simulink model "Simulink_TEP"  (R2024a)
settings: Solver=FixedStepAuto  StartTime=0.0  StopTime=5  FixedStep=1/3600  RelTol=1e-3
model workspace (MAT data in the model file):
  AD : Simulink.Parameter (value not decoded)
  AG : Simulink.Parameter (value not decoded)
  AH : Simulink.Parameter (value not decoded)
  AV : Simulink.Parameter (value not decoded)
  AVP : Simulink.Parameter (value not decoded)
  BCHL : Simulink.Parameter (value not decoded)
  BCHV : Simulink.Parameter (value not decoded)
  BD : Simulink.Parameter (value not decoded)
  BG : Simulink.Parameter (value not decoded)
  BH : Simulink.Parameter (value not decoded)
  BVP : Simulink.Parameter (value not decoded)
  CD : Simulink.Parameter (value not decoded)
  CG : Simulink.Parameter (value not decoded)
  CH : Simulink.Parameter (value not decoded)
  CVP : Simulink.Parameter (value not decoded)
  XMW : Simulink.Parameter (value not decoded)
symbols that are objects in the model workspace (value not decoded): AD, AG, AH, AV, AVP, BD, BG, BH, BVP, CD, CG, CH, CVP, XMW
undefined symbols (not defined in the file or in its folder): magnitude, SETPT, XMEAS, XMV
libraries: mylib x165, dspindex x17
(part 8 of 10)

== system Simulink_TEP/Random number generator/Disturbances I=10-12/TESUB7(11)/Subsystem ==
  In2 : Inport
  G : Inport  Port=2
  If Action Subsystem : Subsystem  TreatAsAtomicUnit=on
  If Action Subsystem1 : Subsystem  TreatAsAtomicUnit=on
  If5 : If  IfExpression=u1 == 0
  Merge : Merge
  G1 : Outport  VectorParamsAs1DForOutWhenUnconnected=off
  wires:
  In2/1 -> If Action Subsystem1/1(In1), If5/1
  If5/2 -> If Action Subsystem1/Action
  If Action Subsystem1/1(Out1) -> Merge/1
  If5/1 -> If Action Subsystem/Action
  If Action Subsystem/1(Out1) -> Merge/2
  G/1 -> If Action Subsystem/1(In1)
  Merge/1 -> G1/1

== system Simulink_TEP/Random number generator/Disturbances I=10-12/TESUB7(11)/TNEXT(11) ==
  Bus Selector : BusSelector  OutputSignals=TNEXT
  Clock3 : Clock
  If3 : If  NumInputs=3  IfExpression=u1 ~= 0 & u1 >= u2 & u3 < 0.1  ShowElse=off
  IF(11) : Outport  VectorParamsAs1DForOutWhenUnconnected=off
  wires:
  Bus Selector/1 -> If3/2  "<TNEXT>"
  Clock3/1 -> If3/1
  If3/1 -> IF(11)/1
  [DIST11] -> Bus Selector/1
  [SWLK_11] -> If3/3

== system Simulink_TEP/Random number generator/Disturbances I=10-12/TESUB7(12)/If Action Subsystem3 ==
  G : Inport
  Action Port : ActionPort  ActionPortLabel=if(u1 ~= 0 & u1 >= u2 & u3 < 0.1)
  Constant : Constant  Value=-1
  TESUB7 G-New : mylib/TESUB7 G-New  SystemSampleTime=-1  VariantActivationTime=update diagram  AllowFlexibleInterface=on  Latency=0  AutoFrameSizeCalculation=off
  TESUB7(12) : Outport  VectorParamsAs1DForOutWhenUnconnected=off
  G_NEW : Outport  Port=2  OutputWhenDisabled=reset  InitialOutput=[0]  VectorParamsAs1DForOutWhenUnconnected=off
  wires:
  Constant/1 -> TESUB7 G-New/1
  G/1 -> TESUB7 G-New/2
  TESUB7 G-New/2 -> G_NEW/1
  TESUB7 G-New/1 -> TESUB7(12)/1

== system Simulink_TEP/Random number generator/Disturbances I=10-12/TESUB7(12)/Subsystem ==
  In2 : Inport
  G : Inport  Port=2
  If Action Subsystem : Subsystem  TreatAsAtomicUnit=on
  If Action Subsystem1 : Subsystem  TreatAsAtomicUnit=on
  If5 : If  IfExpression=u1 == 0
  Merge : Merge
  G1 : Outport  VectorParamsAs1DForOutWhenUnconnected=off
  wires:
  In2/1 -> If Action Subsystem1/1(In1), If5/1
  If5/2 -> If Action Subsystem1/Action
  If Action Subsystem1/1(Out1) -> Merge/1
  If5/1 -> If Action Subsystem/Action
  If Action Subsystem/1(Out1) -> Merge/2
  G/1 -> If Action Subsystem/1(In1)
  Merge/1 -> G1/1

== system Simulink_TEP/Random number generator/Disturbances I=10-12/TESUB7(12)/TNEXT(12) ==
  Bus Selector : BusSelector  OutputSignals=TNEXT
  Clock3 : Clock
  If3 : If  NumInputs=3  IfExpression=u1 ~= 0 & u1 >= u2 & u3 < 0.1  ShowElse=off
  IF(12) : Outport  VectorParamsAs1DForOutWhenUnconnected=off
  wires:
  Bus Selector/1 -> If3/2  "<TNEXT>"
  Clock3/1 -> If3/1
  If3/1 -> IF(12)/1
  [DIST12] -> Bus Selector/1
  [SWLK_12] -> If3/3

== system Simulink_TEP/Random number generator/Process Measurements XMEAS(I) I=1-22/If Action Subsystem3/Subsystem ==
  G : Inport
  Bus Creator : BusCreator  Inputs=5
  Bus Creator1 : BusCreator  Inputs=5
  Bus Creator2 : BusCreator  Inputs=4
  Bus Creator3 : BusCreator  Inputs=5
  Bus Creator4 : BusCreator  Inputs=7
  Subsystem : Subsystem
  Subsystem1 : Subsystem
  Subsystem2 : Subsystem
  Subsystem3 : Subsystem
  XMNS : Outport  VectorParamsAs1DForOutWhenUnconnected=off
  G_NEW : Outport  Port=2  VectorParamsAs1DForOutWhenUnconnected=off
  wires:
  G/1 -> Subsystem/1(G)
  Subsystem/1(XMNS(1)) -> Bus Creator/1
  Subsystem/2(XMNS(2)) -> Bus Creator/2
  Subsystem/3(XMNS(3)) -> Bus Creator/3
  Subsystem/4(XMNS(4)) -> Bus Creator/4
  Subsystem/5(XMNS(5)) -> Bus Creator/5
  Subsystem/6(G_NEW) -> Subsystem1/1(G)
  Subsystem1/6(G_NEW) -> Subsystem2/1(G)
  Subsystem1/2(XMNS(7)) -> Bus Creator1/2
  Subsystem1/3(XMNS(8)) -> Bus Creator1/3
  Subsystem1/4(XMNS(9)) -> Bus Creator1/4
  Subsystem1/1(XMNS(6)) -> Bus Creator1/1
  Subsystem1/5(XMNS(10)) -> Bus Creator1/5
  Bus Creator1/1 -> Bus Creator2/2
  Bus Creator2/1 -> XMNS/1
  Bus Creator/1 -> Bus Creator2/1
  Subsystem2/1(XMNS(11)) -> Bus Creator3/1
  Bus Creator3/1 -> Bus Creator2/3
  Subsystem2/4(XMNS(14)) -> Bus Creator3/4
  Subsystem2/5(XMNS(15)) -> Bus Creator3/5
  Subsystem2/2(XMNS(12)) -> Bus Creator3/2
  Subsystem2/3(XMNS(13)) -> Bus Creator3/3
  Subsystem2/6(G_NEW) -> Subsystem3/1(G)
  Subsystem3/2(XMNS(17)) -> Bus Creator4/2
  Subsystem3/3(XMNS(18)) -> Bus Creator4/3
  Subsystem3/4(XMNS(19)) -> Bus Creator4/4
  Bus Creator4/1 -> Bus Creator2/4
  Subsystem3/5(XMNS(20)) -> Bus Creator4/5
  Subsystem3/8(G_NEW) -> G_NEW/1
  Subsystem3/1(XMNS(16)) -> Bus Creator4/1
  Subsystem3/6(XMNS(21)) -> Bus Creator4/6
  Subsystem3/7(XMNS(22)) -> Bus Creator4/7

== system Simulink_TEP/Random number generator/Process Measurements XMEAS(I) I=1-22/Subsystem/If Action Subsystem ==
  In1 : Inport
  Action Port : ActionPort  ActionPortLabel=if(u1 == 0)
  Out1 : Outport  VectorParamsAs1DForOutWhenUnconnected=off
  wires:
  In1/1 -> Out1/1

== system Simulink_TEP/Random number generator/Process Measurements XMEAS(I) I=1-22/Subsystem/If Action Subsystem1 ==
  In1 : Inport
  Action Port : ActionPort  ActionPortLabel=else
  Out1 : Outport  VectorParamsAs1DForOutWhenUnconnected=off
  wires:
  In1/1 -> Out1/1

== system Simulink_TEP/Random number generator/Process Measurements XMEAS(I) I=23-36/If Action Subsystem3/Subsystem ==
  G : Inport
  Bus Creator : BusCreator  Inputs=5
  Bus Creator1 : BusCreator  Inputs=5
  Bus Creator2 : BusCreator  Inputs=3
  Bus Creator3 : BusCreator  Inputs=4
  Subsystem : Subsystem
  Subsystem1 : Subsystem
  Subsystem2 : Subsystem
  XMNS : Outport  VectorParamsAs1DForOutWhenUnconnected=off
  G_NEW : Outport  Port=2  VectorParamsAs1DForOutWhenUnconnected=off
  wires:
  G/1 -> Subsystem/1(G)
  Subsystem/1(XMNS(23)) -> Bus Creator/1
  Subsystem/2(XMNS(24)) -> Bus Creator/2
  Subsystem/3(XMNS(25)) -> Bus Creator/3
  Subsystem/4(XMNS(26)) -> Bus Creator/4
  Subsystem/5(XMNS(27)) -> Bus Creator/5
  Subsystem/6(G_NEW) -> Subsystem1/1(G)
  Subsystem1/6(G_NEW) -> Subsystem2/1(G)
  Subsystem1/2(XMNS(29)) -> Bus Creator1/2
  Subsystem1/3(XMNS(30)) -> Bus Creator1/3
  Subsystem1/4(XMNS(31)) -> Bus Creator1/4
  Subsystem1/1(XMNS(28)) -> Bus Creator1/1
  Subsystem1/5(XMNS(32)) -> Bus Creator1/5
  Bus Creator1/1 -> Bus Creator2/2
  Bus Creator2/1 -> XMNS/1
  Bus Creator/1 -> Bus Creator2/1
  Subsystem2/1(XMNS(33)) -> Bus Creator3/1
  Bus Creator3/1 -> Bus Creator2/3
  Subsystem2/4(XMNS(36)) -> Bus Creator3/4
  Subsystem2/2(XMNS(34)) -> Bus Creator3/2
  Subsystem2/3(XMNS(35)) -> Bus Creator3/3
  Subsystem2/5(G_NEW) -> G_NEW/1

== system Simulink_TEP/Random number generator/Process Measurements XMEAS(I) I=23-36/Subsystem/If Action Subsystem ==
  In1 : Inport
  Action Port : ActionPort  ActionPortLabel=if(u1 == 0)
  Out1 : Outport  VectorParamsAs1DForOutWhenUnconnected=off
  wires:
  In1/1 -> Out1/1

== system Simulink_TEP/Random number generator/Process Measurements XMEAS(I) I=23-36/Subsystem/If Action Subsystem1 ==
  In1 : Inport
  Action Port : ActionPort  ActionPortLabel=else
  Out1 : Outport  VectorParamsAs1DForOutWhenUnconnected=off
  wires:
  In1/1 -> Out1/1

== system Simulink_TEP/Random number generator/Process Measurements XMEAS(I) I=37-41/If Action Subsystem3/Subsystem ==
  G : Inport
  Bus Creator : BusCreator  Inputs=5
  Subsystem : Subsystem
  XMNS : Outport  VectorParamsAs1DForOutWhenUnconnected=off
  G_NEW : Outport  Port=2  VectorParamsAs1DForOutWhenUnconnected=off
  wires:
  G/1 -> Subsystem/1(G)
  Subsystem/1(XMNS(37)) -> Bus Creator/1
  Subsystem/2(XMNS(38)) -> Bus Creator/2
  Subsystem/3(XMNS(39)) -> Bus Creator/3
  Subsystem/4(XMNS(40)) -> Bus Creator/4
  Subsystem/5(XMNS(41)) -> Bus Creator/5
  Bus Creator/1 -> XMNS/1
  Subsystem/6(G_NEW) -> G_NEW/1

== system Simulink_TEP/Random number generator/Process Measurements XMEAS(I) I=37-41/Subsystem/If Action Subsystem ==
  In1 : Inport
  Action Port : ActionPort  ActionPortLabel=if(u1 == 0)
  Out1 : Outport  VectorParamsAs1DForOutWhenUnconnected=off
  wires:
  In1/1 -> Out1/1

== system Simulink_TEP/Random number generator/Process Measurements XMEAS(I) I=37-41/Subsystem/If Action Subsystem1 ==
  In1 : Inport
  Action Port : ActionPort  ActionPortLabel=else
  Out1 : Outport  VectorParamsAs1DForOutWhenUnconnected=off
  wires:
  In1/1 -> Out1/1

== system Simulink_TEP/Reactor/Reaction Rates/Component reaction rate lb-mol//h/Subsystem ==
  RR : Inport
  " " : Sum  Inputs=---
  Bus Selector : BusSelector  OutputSignals=RR(1),RR(2),RR(3)
  CRXR(1) : Outport  VectorParamsAs1DForOutWhenUnconnected=off
  wires:
  " "/1 -> CRXR(1)/1  "CRXR(1)"
  Bus Selector/2 -> " "/2  "<RR(2)>"
  Bus Selector/3 -> " "/3  "<RR(3)>"
  RR/1 -> Bus Selector/1
  Bus Selector/1 -> " "/1  "<RR(1)>"

== system Simulink_TEP/Reactor/Reaction Rates/Component reaction rate lb-mol//h/Subsystem1 ==
  RR : Inport
  " " : Sum  Inputs=--
  Bus Selector : BusSelector  OutputSignals=RR(1),RR(2)
  CRXR(3) : Outport  VectorParamsAs1DForOutWhenUnconnected=off
  wires:
  " "/1 -> CRXR(3)/1  "CRXR(3)"
  RR/1 -> Bus Selector/1
  Bus Selector/1 -> " "/1  "<RR(1)>"
  Bus Selector/2 -> " "/2  "<RR(2)>"

== system Simulink_TEP/Reactor/Reaction Rates/Component reaction rate lb-mol//h/Subsystem2 ==
  RR : Inport
  " " : Sum  Inputs=--
  Bus Selector : BusSelector  OutputSignals=RR(1),RR(4)
  Gain : Gain  Gain=1.5
  CRXR(4) : Outport  VectorParamsAs1DForOutWhenUnconnected=off
  wires:
  Gain/1 -> " "/2
  Bus Selector/1 -> " "/1  "<RR(1)>"
  " "/1 -> CRXR(4)/1  "CRXR(4)"
  RR/1 -> Bus Selector/1
  Bus Selector/2 -> Gain/1  "<RR(4)>"

== system Simulink_TEP/Reactor/Reaction Rates/Component reaction rate lb-mol//h/Subsystem3 ==
  RR : Inport
  " " : Sum  Inputs=--
  Bus Selector : BusSelector  OutputSignals=RR(2),RR(3)
  CRXR(5) : Outport  VectorParamsAs1DForOutWhenUnconnected=off
  wires:
  " "/1 -> CRXR(5)/1  "CRXR(5)"
  RR/1 -> Bus Selector/1
  Bus Selector/1 -> " "/1  "<RR(2)>"
  Bus Selector/2 -> " "/2  "<RR(3)>"

== system Simulink_TEP/Reactor/Reaction Rates/Component reaction rate lb-mol//h/Subsystem4 ==
  RR : Inport
  " " : Sum
  Bus Selector : BusSelector  OutputSignals=RR(3),RR(4)
  CRXR(6) : Outport  VectorParamsAs1DForOutWhenUnconnected=off
  wires:
  " "/1 -> CRXR(6)/1  "CRXR(6)"
  RR/1 -> Bus Selector/1
  Bus Selector/2 -> " "/2  "<RR(4)>"
  Bus Selector/1 -> " "/1  "<RR(3)>"

== system Simulink_TEP/Reactor/Reaction Rates/Component reaction rate lb-mol//h/Subsystem5 ==
  RR : Inport
  Bus Selector : BusSelector  OutputSignals=RR(1)
  Gain : Gain
  CRXR(7) : Outport  VectorParamsAs1DForOutWhenUnconnected=off
  wires:
  Bus Selector/1 -> Gain/1  "<RR(1)>"
  RR/1 -> Bus Selector/1
  Gain/1 -> CRXR(7)/1  "CRXR(7)"

== system Simulink_TEP/Reactor/Reaction Rates/Component reaction rate lb-mol//h/Subsystem6 ==
  RR : Inport
  " " : Gain
  Bus Selector : BusSelector  OutputSignals=RR(2)
  CRXR(8) : Outport  VectorParamsAs1DForOutWhenUnconnected=off
  wires:
  " "/1 -> CRXR(8)/1  "CRXR(8)"
  RR/1 -> Bus Selector/1
  Bus Selector/1 -> " "/1  "<RR(2)>"

== system Simulink_TEP/Reactor/Reaction Rates/Reaction rates lb-mol//h/ Reaction rate of reaction 4 lb-mol//ft3·h     ==
  PPR : Inport
  TKR : Inport  Port=2
  Activation energy cal/mol : Constant  Value=60000
  Bus Selector : BusSelector  OutputSignals=PPR(1),PPR(4)
  Divide : Product  Inputs=*//
  Divide1 : Product  Inputs=3
  Gain : Gain  Gain=0.767488334
  Math Function2 : Math  SignedPower=on
  Preexponential factor lb-mol/ft3·h·mmHg : Constant  Value=53.4060443
  Subtract : Sum  Inputs=+-
  Universal gas constant cal/mol·K : Constant  Value=1.987
  RR(4) : Outport  VectorParamsAs1DForOutWhenUnconnected=off
  wires:
  Divide/1 -> Subtract/2
  Universal gas constant cal/mol·K/1 -> Divide/2
  Preexponential factor lb-mol/ft3·h·mmHg/1 -> Subtract/1
  Activation energy cal/mol/1 -> Divide/1
  TKR/1 -> Divide/3
  Subtract/1 -> Math Function2/1
  Divide1/1 -> RR(4)/1
  Bus Selector/2 -> Divide1/3  "<PPR(4)>"
  Gain/1 -> Divide1/1
  Math Function2/1 -> Gain/1
  PPR/1 -> Bus Selector/1
  Bus Selector/1 -> Divide1/2  "<PPR(1)>"

== system Simulink_TEP/Reactor/Reaction Rates/Reaction rates lb-mol//h/Reaction rate of reaction 1 lb-mol//ft3·h ==
  PPR : Inport
  TKR : Inport  Port=2
  " " : Constant  Value=0
  Abs : Abs  SaturateOnIntegerOverflow=off
  Bus Selector : BusSelector  OutputSignals=PPR(1),PPR(3)
  If : If  NumInputs=2  IfExpression=u1>0 & u2>0
  If Action Subsystem : Subsystem  TreatAsAtomicUnit=on
  If Action Subsystem2 : Subsystem  TreatAsAtomicUnit=on
  Merge1 : Merge
  "RR(1) Reaction rate of 1st reaction lb-mol/ft3·h " : Subsystem
  RR(1) : Outport  VectorParamsAs1DForOutWhenUnconnected=off
  wires:
  "RR(1) Reaction rate of 1st reaction lb-mol/ft3·h "/1(RR(1)) -> If Action Subsystem/1(In1)
  If/1 -> If Action Subsystem/Action
  " "/1 -> If Action Subsystem2/1(In1)
  If/2 -> If Action Subsystem2/Action
  Merge1/1 -> Abs/1
  If Action Subsystem/1(Out1) -> Merge1/1
  If Action Subsystem2/1(Out1) -> Merge1/2
  TKR/1 -> "RR(1) Reaction rate of 1st reaction lb-mol/ft3·h "/2(TKR)
  Abs/1 -> RR(1)/1
  PPR/1 -> "RR(1) Reaction rate of 1st reaction lb-mol/ft3·h "/1(PPR), Bus Selector/1
  Bus Selector/1 -> If/1  "<PPR(1)>"
  Bus Selector/2 -> If/2  "<PPR(3)>"

== system Simulink_TEP/Reactor/Reaction Rates/Reaction rates lb-mol//h/Reaction rate of reaction 2 lb-mol//ft3·h ==
  PPR : Inport
  TKR : Inport  Port=2
  " " : Constant  Value=0
  Abs : Abs  SaturateOnIntegerOverflow=off
  Bus Selector : BusSelector  OutputSignals=PPR(1),PPR(3)
  If : If  NumInputs=2  IfExpression=u1>0 & u2>0
  If Action Subsystem : Subsystem  TreatAsAtomicUnit=on
  If Action Subsystem2 : Subsystem  TreatAsAtomicUnit=on
  Merge1 : Merge
  "RR(2) Reaction rate of 2nd reaction lb-mol/ft3·h " : Subsystem
  RR(2) : Outport  VectorParamsAs1DForOutWhenUnconnected=off
  wires:
  If/1 -> If Action Subsystem/Action
  If/2 -> If Action Subsystem2/Action
  "RR(2) Reaction rate of 2nd reaction lb-mol/ft3·h "/1(RR(2)) -> If Action Subsystem/1(In1)
  " "/1 -> If Action Subsystem2/1(In1)
  If Action Subsystem2/1(Out1) -> Merge1/2
  TKR/1 -> "RR(2) Reaction rate of 2nd reaction lb-mol/ft3·h "/2(TKR)
  If Action Subsystem/1(Out1) -> Merge1/1
  Merge1/1 -> Abs/1
  Abs/1 -> RR(2)/1
  PPR/1 -> "RR(2) Reaction rate of 2nd reaction lb-mol/ft3·h "/1(PPR), Bus Selector/1
  Bus Selector/1 -> If/1  "<PPR(1)>"
  Bus Selector/2 -> If/2  "<PPR(3)>"

== system Simulink_TEP/Reactor/Reaction Rates/Reaction rates lb-mol//h/Reaction rate of reaction 3 lb-mol//ft3·h   ==
  PPR : Inport
  TKR : Inport  Port=2
  Activation energy cal/mol : Constant  Value=60000
  Bus Selector : BusSelector  OutputSignals=PPR(1),PPR(5)
  Divide : Product  Inputs=*//
  Divide1 : Product  Inputs=3
  Math Function2 : Math  SignedPower=on
  Preexponential factor lb-mol/ft3·h·mmHg : Constant  Value=53.4060443
  Subtract : Sum  Inputs=+-
  Universal gas constant cal/mol·K : Constant  Value=1.987
  RR(3) : Outport  VectorParamsAs1DForOutWhenUnconnected=off
  wires:
  Divide/1 -> Subtract/2
  Universal gas constant cal/mol·K/1 -> Divide/2
  Preexponential factor lb-mol/ft3·h·mmHg/1 -> Subtract/1
  Activation energy cal/mol/1 -> Divide/1
  TKR/1 -> Divide/3
  Subtract/1 -> Math Function2/1
  Bus Selector/2 -> Divide1/3  "<PPR(5)>"
  Divide1/1 -> RR(3)/1
  Math Function2/1 -> Divide1/1
  PPR/1 -> Bus Selector/1
  Bus Selector/1 -> Divide1/2  "<PPR(1)>"

== system Simulink_TEP/Reactor/Reactor Heat exchanger/Position of Valve 12 %/Control valve ==
  XMV(12) : Inport
  Valve opening limits : mylib/Valve opening limits  SystemSampleTime=-1  VariantActivationTime=update diagram  AllowFlexibleInterface=on  Latency=0  AutoFrameSizeCalculation=off
  VCV(12) : Outport  PortDimensions=1  VectorParamsAs1DForOutWhenUnconnected=off
  wires:
  Valve opening limits/1 -> VCV(12)/1
  XMV(12)/1 -> Valve opening limits/1

== system Simulink_TEP/Reactor/Reactor Heat exchanger/Reactor Heat exchanger/AGSP Agitation speed ==
  VPOS(12) : Inport
  " " : Product  Inputs=*/
  Add : Sum
  Constant1 : Constant  Value=150
  Constant2 : Constant  Value=100
  AGSP : Outport  VectorParamsAs1DForOutWhenUnconnected=off
  wires:
  Constant2/1 -> " "/2
  " "/1 -> AGSP/1
  VPOS(12)/1 -> Add/1
  Constant1/1 -> Add/2
  Add/1 -> " "/1

== system Simulink_TEP/Reactor/Reactor Heat exchanger/Reactor Heat exchanger/FWR Flow of cooling water to reactor lb-mol//h ==
  VPOS(10) : Inport
  VRNG(10) : Inport  Port=2
  " " : Product  Inputs=**/
  Constant2 : Constant  Value=100
  FWR : Outport  VectorParamsAs1DForOutWhenUnconnected=off
  wires:
  Constant2/1 -> " "/3
  " "/1 -> FWR/1
  VPOS(10)/1 -> " "/1
  VRNG(10)/1 -> " "/2

== system Simulink_TEP/Reactor/Reactor Heat exchanger/Reactor Heat exchanger/Subsystem ==
  VLR : Inport
  Constant : Constant  Value=7.8
  Constant1 : Constant
  Constant2 : Constant  Value=0
  Constant3 : Constant  Value=0.025
  Constant4 : Constant  Value=0.25
  Divide : Product  Inputs=*/
  Divide1 : Product  Inputs=**
  If : If  IfExpression=u1 > 50  ElseIfExpressions=u1 < 10
  If Action Subsystem : Subsystem  TreatAsAtomicUnit=on
  If Action Subsystem1 : Subsystem  TreatAsAtomicUnit=on
  If Action Subsystem2 : Subsystem  TreatAsAtomicUnit=on
  Subtract : Sum  Inputs=+-
  UARLEV : Merge  Inputs=3
  "UARLEV " : Outport  VectorParamsAs1DForOutWhenUnconnected=off
  wires:
  If/2 -> If Action Subsystem1/Action
  If/1 -> If Action Subsystem/Action
  UARLEV/1 -> "UARLEV "/1
  If Action Subsystem1/1(Out1) -> UARLEV/2
  If Action Subsystem/1(Out1) -> UARLEV/1
  If/3 -> If Action Subsystem2/Action
  If Action Subsystem2/1(Out1) -> UARLEV/3
  VLR/1 -> Divide/1
  Constant/1 -> Divide/2
  Divide/1 -> Divide1/2, If/1
  Constant1/1 -> If Action Subsystem/1(In1)
  Constant2/1 -> If Action Subsystem1/1(In1)
  Constant3/1 -> Divide1/1
  Divide1/1 -> Subtract/1
  Constant4/1 -> Subtract/2
  Subtract/1 -> If Action Subsystem2/1(In1)

== system Simulink_TEP/Reactor/Reactor Heat exchanger/Reactor Heat exchanger/Subsystem1 ==
  FWR : Inport
  QUR : Inport  Port=2  PortDimensions=1
  Constant1 : Constant  Value=1e6
  Constant2 : Constant  Value=1.8
  Constant6 : Constant  Value=500.53
  Divide : Product  Inputs=*/
  Divide1 : Product
  Divide2 : Product  Inputs=*/
  HWR : Constant  Value=7060
  Product : Product  Inputs=3
  Subtract : Sum  Inputs=+-
  TCWR : Subsystem
  TCWR-TWR : Sum  Inputs=+-
  YP(37) : Integrator  InitialConditionSource=external
  YY(37) : Constant  Value=94.59927549
  "YY(37) " : Outport  VectorParamsAs1DForOutWhenUnconnected=off
  tag scope: TWR=global
  wires:
  Divide2/1 -> YP(37)/1
  YY(37)/1 -> YP(37)/2
  TCWR/1(TCWR) -> TCWR-TWR/1
  YP(37)/1 -> [TWR], "YY(37) "/1, TCWR-TWR/2
  FWR/1 -> Product/1
  Constant6/1 -> Product/2
  TCWR-TWR/1 -> Product/3
  QUR/1 -> Divide1/1
  Constant1/1 -> Divide1/2
  Divide1/1 -> Divide/1
  Constant2/1 -> Divide/2
  Product/1 -> Subtract/1
  Divide/1 -> Subtract/2
  Subtract/1 -> Divide2/1
  HWR/1 -> Divide2/2

== system Simulink_TEP/Reactor/Stream 8/Subsystem/If Action Subsystem ==
  In1 : Inport
  Action Port : ActionPort  ActionPortLabel=if(u1 < 0)
  Out1 : Outport  VectorParamsAs1DForOutWhenUnconnected=off
  wires:
  In1/1 -> Out1/1

== system Simulink_TEP/Reactor/Stream 8/Subsystem/If Action Subsystem1 ==
  In1 : Inport
  Action Port : ActionPort  ActionPortLabel=else
  Out1 : Outport  VectorParamsAs1DForOutWhenUnconnected=off
  wires:
  In1/1 -> Out1/1

== system Simulink_TEP/Reactor/Volume of Reactor/DLR Molar Density of Liquids in Reactor lb-mol//ft³    /DLR Molar Density of Liquids in Reactor lb-mol//ft³  ==
  X : Inport
  T : Inport  Port=2
  "  " : Constant
  "    " : Product  Inputs=*/
  AD(I) : Constant  Value=AD
  Add2 : Sum
  BD(I) : Constant  Value=BD
  CD(I) : Constant  Value=CD
  Liquid Density of Components lb/ft³ : Sum
  Molecular weight of components lb/lb-mol : Constant  Value=XMW
  Product : Product
  Product1 : Product
  Product2 : Product
  Sum of Elements : Sum  Inputs=+
  V Molar Volume of Components ft³/lb-mol : Product  Inputs=*/
  "R " : Outport  VectorParamsAs1DForOutWhenUnconnected=off
  wires:
  Liquid Density of Components lb/ft³/1 -> V Molar Volume of Components ft³/lb-mol/2
  Product1/1 -> Liquid Density of Components lb/ft³/2
  T/1 -> Product1/2, Product/2
  "  "/1 -> "    "/1
  AD(I)/1 -> Liquid Density of Components lb/ft³/1
  Add2/1 -> Product1/1
  V Molar Volume of Components ft³/lb-mol/1 -> Sum of Elements/1
  CD(I)/1 -> Product/1
  Product2/1 -> V Molar Volume of Components ft³/lb-mol/1
  BD(I)/1 -> Add2/1
  Product/1 -> Add2/2
  "    "/1 -> "R "/1
  X/1 -> Product2/1
  Sum of Elements/1 -> "    "/2
  Molecular weight of components lb/lb-mol/1 -> Product2/2

== system Simulink_TEP/Separator/Stream 10/Subsystem/If Action Subsystem ==
  In1 : Inport
  Action Port : ActionPort  ActionPortLabel=if(u1 < 0)
  Out1 : Outport  VectorParamsAs1DForOutWhenUnconnected=off
  wires:
  In1/1 -> Out1/1

== system Simulink_TEP/Separator/Stream 10/Subsystem/If Action Subsystem1 ==
  In1 : Inport
  Action Port : ActionPort  ActionPortLabel=else
  Out1 : Outport  VectorParamsAs1DForOutWhenUnconnected=off
  wires:
  In1/1 -> Out1/1

== system Simulink_TEP/Separator/Stream 9/Subsystem/If Action Subsystem2 ==
  In1 : Inport
  Action Port : ActionPort  ActionPortLabel=if(u1 < 1E-3)
  Out1 : Outport  VectorParamsAs1DForOutWhenUnconnected=off
  wires:
  In1/1 -> Out1/1

== system Simulink_TEP/Separator/Stream 9/Subsystem/If Action Subsystem3 ==
  In1 : Inport
  Action Port : ActionPort  ActionPortLabel=else
  Out1 : Outport  PortDimensions=1  VectorParamsAs1DForOutWhenUnconnected=off
  wires:
  In1/1 -> Out1/1

== system Simulink_TEP/Separator/Stream 9/Subsystem/Pressure drop ==
  Constant : Constant  Value=0.0
  DLP : Sum  Inputs=+-
  DLP Pressure drop between separator and reactor : Merge
  If : If  IfExpression=u1 < 0
  If Action Subsystem : Subsystem  TreatAsAtomicUnit=on
  If Action Subsystem1 : Subsystem  TreatAsAtomicUnit=on
  Out1 : Outport  VectorParamsAs1DForOutWhenUnconnected=off
  wires:
  DLP Pressure drop between separator and reactor/1 -> Out1/1
  [PTV] -> DLP/1
  Constant/1 -> If Action Subsystem/1(In1)
  DLP/1 -> If Action Subsystem1/1(In1), If/1
  If/2 -> If Action Subsystem1/Action
  If/1 -> If Action Subsystem/Action
  [PTS] -> DLP/2
  If Action Subsystem1/1(Out1) -> DLP Pressure drop between separator and reactor/2
  If Action Subsystem/1(Out1) -> DLP Pressure drop between separator and reactor/1

== system Simulink_TEP/Separator/Volume of Separator/DLS Molar Density of Liquids in Reactor lb-mol//ft³    /DLS Molar Density of Liquids in Separator lb-mol//ft³  ==
  X : Inport
  T : Inport  Port=2
  "  " : Constant
  "    " : Product  Inputs=*/
  AD(I) : Constant  Value=AD
  Add2 : Sum
  BD(I) : Constant  Value=BD
  CD(I) : Constant  Value=CD
  Display : Display
  Display1 : Display
  Display2 : Display
  Liquid Density of Components lb/ft³ : Sum
  Product : Product
  Product1 : Product
  Product2 : Product
  Sum of Elements : Sum  Inputs=+
  V Molar Volume of Components ft³/lb-mol : Product  Inputs=*/
  XMW : Constant  Value=XMW
  "R " : Outport  VectorParamsAs1DForOutWhenUnconnected=off
  wires:
  Liquid Density of Components lb/ft³/1 -> V Molar Volume of Components ft³/lb-mol/2
  Product1/1 -> Liquid Density of Components lb/ft³/2
  T/1 -> Display/1, Product1/2, Product/2
  "  "/1 -> "    "/1
  AD(I)/1 -> Liquid Density of Components lb/ft³/1
  Add2/1 -> Product1/1
  V Molar Volume of Components ft³/lb-mol/1 -> Sum of Elements/1
  CD(I)/1 -> Product/1
  Product2/1 -> V Molar Volume of Components ft³/lb-mol/1
  BD(I)/1 -> Add2/1
  Product/1 -> Add2/2
  "    "/1 -> Display1/1, "R "/1
  X/1 -> Display2/1, Product2/1
  Sum of Elements/1 -> "    "/2
  XMW/1 -> Product2/2

== system Simulink_TEP/Stripper/Split Fractions/Split fraction/If Action Subsystem ==
  In1 : Inport
  Action Port : ActionPort  ActionPortLabel=if(u1 >0.1)
  Out1 : Outport  VectorParamsAs1DForOutWhenUnconnected=off
  wires:
  In1/1 -> Out1/1

== system Simulink_TEP/Stripper/Split Fractions/Split fraction/If Action Subsystem1 ==
  In1 : Inport
  Action Port : ActionPort  ActionPortLabel=if(u1 >170)
  Out1 : Outport  VectorParamsAs1DForOutWhenUnconnected=off
  wires:
  In1/1 -> Out1/1

== system Simulink_TEP/Stripper/Split Fractions/Split fraction/If Action Subsystem2 ==
  In1 : Inport
  Action Port : ActionPort  ActionPortLabel=elseif(u1<5.292)
  Out1 : Outport  VectorParamsAs1DForOutWhenUnconnected=off
  wires:
  In1/1 -> Out1/1

== system Simulink_TEP/Stripper/Split Fractions/Split fraction/If Action Subsystem3 ==
  In1 : Inport
  Action Port : ActionPort  ActionPortLabel=else
  Out1 : Outport  VectorParamsAs1DForOutWhenUnconnected=off
  wires:
  In1/1 -> Out1/1

== system Simulink_TEP/Stripper/Split Fractions/Split fraction/If Action Subsystem4 ==
  In1 : Inport
  Action Port : ActionPort  ActionPortLabel=else
  Out1 : Outport  VectorParamsAs1DForOutWhenUnconnected=off
  wires:
  In1/1 -> Out1/1

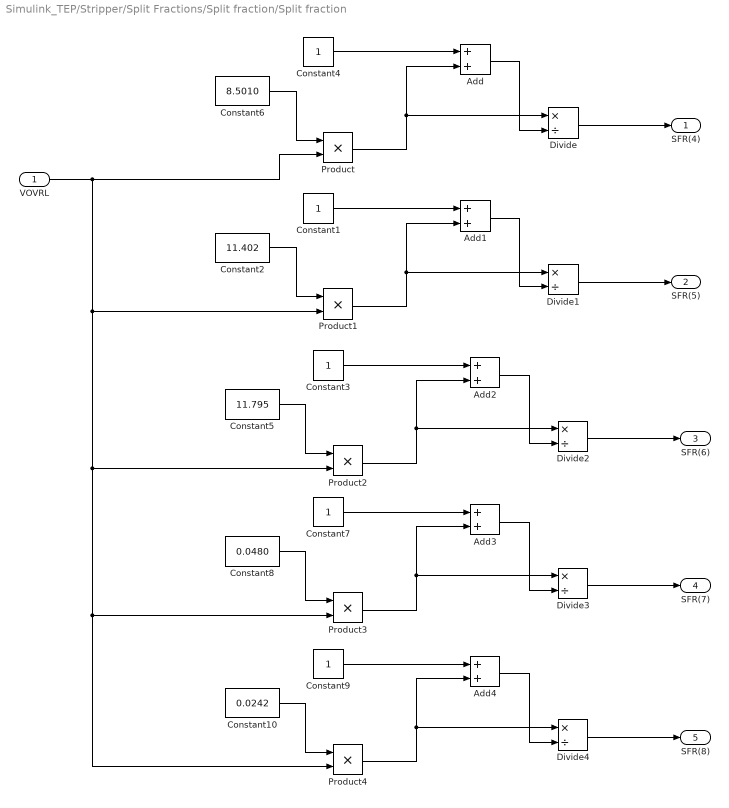
== system Simulink_TEP/Stripper/Split Fractions/Split fraction/Split fraction ==
  VOVRL : Inport
  Add{,1..4} (5 alike) : Sum
  Constant{1,3..4,7,9} (5 alike) : Constant
  Constant10 : Constant  Value=0.0242
  Constant2 : Constant  Value=11.402
  Constant5 : Constant  Value=11.795
  Constant6 : Constant  Value=8.5010
  Constant8 : Constant  Value=0.0480
  Divide{,1..4} (5 alike) : Product  Inputs=*/
  Product{,1..4} (5 alike) : Product
  SFR(4) : Outport  PortDimensions=1  VectorParamsAs1DForOutWhenUnconnected=off
  SFR(5) : Outport  Port=2  PortDimensions=1  VectorParamsAs1DForOutWhenUnconnected=off
  SFR(6) : Outport  Port=3  PortDimensions=1  VectorParamsAs1DForOutWhenUnconnected=off
  SFR(7) : Outport  Port=4  PortDimensions=1  VectorParamsAs1DForOutWhenUnconnected=off
  SFR(8) : Outport  Port=5  PortDimensions=1  VectorParamsAs1DForOutWhenUnconnected=off
  wires:
  Add/1 -> Divide/2
  Product/1 -> Divide/1, Add/2
  Constant4/1 -> Add/1
  Constant6/1 -> Product/1
  Divide/1 -> SFR(4)/1
  Product1/1 -> Divide1/1, Add1/2
  Add1/1 -> Divide1/2
  Constant1/1 -> Add1/1
  Constant2/1 -> Product1/1
  Divide1/1 -> SFR(5)/1
  Divide2/1 -> SFR(6)/1
  Product2/1 -> Divide2/1, Add2/2
  Add2/1 -> Divide2/2
  Constant3/1 -> Add2/1
  Constant5/1 -> Product2/1
  Divide3/1 -> SFR(7)/1
  Product3/1 -> Divide3/1, Add3/2
  Add3/1 -> Divide3/2
  Constant7/1 -> Add3/1
  Constant8/1 -> Product3/1
  Divide4/1 -> SFR(8)/1
  Product4/1 -> Divide4/1, Add4/2
  VOVRL/1 -> Product4/2, Product3/2, Product2/2, Product1/2, Product/2
  Add4/1 -> Divide4/2
  Constant9/1 -> Add4/1
  Constant10/1 -> Product4/1

== system Simulink_TEP/Stripper/Volume of Stripper/DLC Molar Density of Liquids in Stripper lb-mol//ft³    /DLC Molar Density of Liquids in Stripper lb-mol//ft³  ==
  X : Inport
  T : Inport  Port=2
  "  " : Constant
  "    " : Product  Inputs=*/
  AD(I) : Constant  Value=AD
  Add2 : Sum
  BD(I) : Constant  Value=BD
  CD(I) : Constant  Value=CD
  Constant : Constant  Value=XMW
  Liquid Density of Components lb/ft³ : Sum
  Product : Product
  Product1 : Product
  Product2 : Product
  Sum of Elements : Sum  Inputs=+
  V Molar Volume of Components ft³/lb-mol : Product  Inputs=*/
  "R " : Outport  VectorParamsAs1DForOutWhenUnconnected=off
  wires:
  Liquid Density of Components lb/ft³/1 -> V Molar Volume of Components ft³/lb-mol/2
  Product1/1 -> Liquid Density of Components lb/ft³/2
  T/1 -> Product1/2, Product/2
  "  "/1 -> "    "/1
  AD(I)/1 -> Liquid Density of Components lb/ft³/1
  Add2/1 -> Product1/1
  V Molar Volume of Components ft³/lb-mol/1 -> Sum of Elements/1
  CD(I)/1 -> Product/1
  Product2/1 -> V Molar Volume of Components ft³/lb-mol/1
  BD(I)/1 -> Add2/1
  Product/1 -> Add2/2
  "    "/1 -> "R "/1
  X/1 -> Product2/1
  Sum of Elements/1 -> "    "/2
  Constant/1 -> Product2/2

== system Simulink_TEP/Subsystem/Braatz/ /CONTROL 1 ==
  XMEAS(2) : Inport
  SETPT(1) : Inport  Port=2
  Constant1 : Constant  Value=GAIN1
  Constant2 : Constant  Value=HIGH1
  Constant3 : Constant  Value=SI1
  P Control : mylib/Braatz Control/P Control  SystemSampleTime=-1  VariantActivationTime=update diagram  AllowFlexibleInterface=on  Latency=0  AutoFrameSizeCalculation=off
  Sampling interval : mylib/Braatz Control/Sampling interval  SystemSampleTime=-1  VariantActivationTime=update diagram  AllowFlexibleInterface=on  Latency=0  AutoFrameSizeCalculation=off
  Unit Delay : UnitDelay  InitialCondition=XMV1_0  SampleTime=-1  HasFrameUpgradeWarning=on
  Unit Delay1 : UnitDelay  SampleTime=-1  HasFrameUpgradeWarning=on
  XMV(1) : Outport  VectorParamsAs1DForOutWhenUnconnected=off
  wires:
  Constant2/1 -> P Control/5
  Constant1/1 -> P Control/3
  SETPT(1)/1 -> P Control/1
  Unit Delay/1 -> P Control/2
  XMEAS(2)/1 -> P Control/4
  P Control/1 -> XMV(1)/1, Unit Delay/1
  Sampling interval/1 -> P Control/Action
  Constant3/1 -> Sampling interval/1
  Unit Delay1/1 -> P Control/6
  P Control/2 -> Unit Delay1/1

== system Simulink_TEP/Subsystem/Braatz/ /CONTROL 14 ==
  XMEAS(26) : Inport
  Constant : Constant  Value=SETPT14
  Constant1 : Constant  Value=GAIN14
  Constant2 : Constant  Value=TAUI14
  Constant3 : Constant  Value=HIGH14
  Constant5 : Constant  Value=SI14
  Constant6 : Constant  Value=HIGH1
  PI Control Setpoint : mylib/Braatz Control/PI Control Setpoint  SystemSampleTime=-1  VariantActivationTime=update diagram  AllowFlexibleInterface=on  Latency=0  AutoFrameSizeCalculation=off
  Sampling interval : mylib/Braatz Control/Sampling interval  SystemSampleTime=-1  VariantActivationTime=update diagram  AllowFlexibleInterface=on  Latency=0  AutoFrameSizeCalculation=off
  Unit Delay : UnitDelay  InitialCondition=SETPT1  SampleTime=-1  HasFrameUpgradeWarning=on
  Unit Delay1 : UnitDelay  SampleTime=-1  HasFrameUpgradeWarning=on
  SETPT(1) : Outport  VectorParamsAs1DForOutWhenUnconnected=off
  wires:
  Sampling interval/1 -> PI Control Setpoint/Action
  Constant/1 -> PI Control Setpoint/1
  XMEAS(26)/1 -> PI Control Setpoint/2
  PI Control Setpoint/1 -> SETPT(1)/1, Unit Delay/1
  Constant2/1 -> PI Control Setpoint/8
  Constant5/1 -> PI Control Setpoint/7, Sampling interval/1
  Constant1/1 -> PI Control Setpoint/6
  Constant3/1 -> PI Control Setpoint/3
  Unit Delay/1 -> PI Control Setpoint/4
  Constant6/1 -> PI Control Setpoint/5
  PI Control Setpoint/2 -> Unit Delay1/1
  Unit Delay1/1 -> PI Control Setpoint/9

== system Simulink_TEP/Subsystem/Braatz/ 1/CONTROL 15 ==
  XMEAS(27) : Inport
  Constant : Constant  Value=SETPT15
  Constant1 : Constant  Value=GAIN15
  Constant2 : Constant  Value=TAUI15
  Constant3 : Constant  Value=HIGH15
  Constant5 : Constant  Value=SI15
  Constant6 : Constant  Value=HIGH2
  PI Control Setpoint : mylib/Braatz Control/PI Control Setpoint  SystemSampleTime=-1  VariantActivationTime=update diagram  AllowFlexibleInterface=on  Latency=0  AutoFrameSizeCalculation=off
  Sampling interval : mylib/Braatz Control/Sampling interval  SystemSampleTime=-1  VariantActivationTime=update diagram  AllowFlexibleInterface=on  Latency=0  AutoFrameSizeCalculation=off
  Unit Delay : UnitDelay  InitialCondition=SETPT2  SampleTime=-1  HasFrameUpgradeWarning=on
  Unit Delay1 : UnitDelay  SampleTime=-1  HasFrameUpgradeWarning=on
  SETPT(2) : Outport  VectorParamsAs1DForOutWhenUnconnected=off
  wires:
  Sampling interval/1 -> PI Control Setpoint/Action
  Constant/1 -> PI Control Setpoint/1
  XMEAS(27)/1 -> PI Control Setpoint/2
  PI Control Setpoint/1 -> SETPT(2)/1, Unit Delay/1
  Constant2/1 -> PI Control Setpoint/8
  Constant5/1 -> PI Control Setpoint/7, Sampling interval/1
  Constant1/1 -> PI Control Setpoint/6
  Constant3/1 -> PI Control Setpoint/3
  Unit Delay/1 -> PI Control Setpoint/4
  Constant6/1 -> PI Control Setpoint/5
  PI Control Setpoint/2 -> Unit Delay1/1
  Unit Delay1/1 -> PI Control Setpoint/9

== system Simulink_TEP/Subsystem/Braatz/ 1/CONTROL 2 ==
  XMEAS(2) : Inport
  SETPT(2) : Inport  Port=2
  Constant1 : Constant  Value=GAIN2
  Constant2 : Constant  Value=HIGH2
  Constant3 : Constant  Value=SI2
  P Control : mylib/Braatz Control/P Control  SystemSampleTime=-1  VariantActivationTime=update diagram  AllowFlexibleInterface=on  Latency=0  AutoFrameSizeCalculation=off
  Sampling interval : mylib/Braatz Control/Sampling interval  SystemSampleTime=-1  VariantActivationTime=update diagram  AllowFlexibleInterface=on  Latency=0  AutoFrameSizeCalculation=off
  Unit Delay : UnitDelay  InitialCondition=XMV2_0  SampleTime=-1  HasFrameUpgradeWarning=on
  Unit Delay1 : UnitDelay  SampleTime=-1  HasFrameUpgradeWarning=on
  XMV(2) : Outport  VectorParamsAs1DForOutWhenUnconnected=off
  wires:
  Constant2/1 -> P Control/5
  Constant1/1 -> P Control/3
  SETPT(2)/1 -> P Control/1
  Unit Delay/1 -> P Control/2
  XMEAS(2)/1 -> P Control/4
  P Control/1 -> XMV(2)/1, Unit Delay/1
  Sampling interval/1 -> P Control/Action
  Constant3/1 -> Sampling interval/1
  P Control/2 -> Unit Delay1/1
  Unit Delay1/1 -> P Control/6

== system Simulink_TEP/Subsystem/Braatz/ 10/CONTROL 19 ==
  XMEAS(30) : Inport
  Constant : Constant  Value=SETPT19
  Constant1 : Constant  Value=GAIN19
  Constant2 : Constant  Value=TAUI19
  Constant3 : Constant  Value=HIGH19
  Constant5 : Constant  Value=SI19
  Constant6 : Constant  Value=HIGH6
  PI Control Setpoint : mylib/Braatz Control/PI Control Setpoint  SystemSampleTime=-1  VariantActivationTime=update diagram  AllowFlexibleInterface=on  Latency=0  AutoFrameSizeCalculation=off
  Sampling interval : mylib/Braatz Control/Sampling interval  SystemSampleTime=-1  VariantActivationTime=update diagram  AllowFlexibleInterface=on  Latency=0  AutoFrameSizeCalculation=off
  Unit Delay : UnitDelay  InitialCondition=SETPT6  SampleTime=-1  HasFrameUpgradeWarning=on
  Unit Delay1 : UnitDelay  SampleTime=-1  HasFrameUpgradeWarning=on
  SETPT(6) : Outport  VectorParamsAs1DForOutWhenUnconnected=off
  wires:
  Sampling interval/1 -> PI Control Setpoint/Action
  Constant/1 -> PI Control Setpoint/1
  XMEAS(30)/1 -> PI Control Setpoint/2
  PI Control Setpoint/1 -> SETPT(6)/1, Unit Delay/1
  Constant2/1 -> PI Control Setpoint/8
  Constant5/1 -> PI Control Setpoint/7, Sampling interval/1
  Constant1/1 -> PI Control Setpoint/6
  Constant3/1 -> PI Control Setpoint/3
  Unit Delay/1 -> PI Control Setpoint/4
  Constant6/1 -> PI Control Setpoint/5
  PI Control Setpoint/2 -> Unit Delay1/1
  Unit Delay1/1 -> PI Control Setpoint/9

== system Simulink_TEP/Subsystem/Braatz/ 10/CONTROL 6 ==
  SETPT(6) : Inport
  XMEAS : Inport  Port=2
  Constant1 : Constant  Value=GAIN6
  Constant2 : Constant  Value=HIGH6
  Constant3 : Constant  Value=SI6
  P Control : Subsystem
  Sampling interval : mylib/Braatz Control/Sampling interval  SystemSampleTime=-1  VariantActivationTime=update diagram  AllowFlexibleInterface=on  Latency=0  AutoFrameSizeCalculation=off
  Unit Delay : UnitDelay  InitialCondition=XMV6_0  SampleTime=-1  HasFrameUpgradeWarning=on
  XMV(6) : Outport  VectorParamsAs1DForOutWhenUnconnected=off
  wires:
  Constant2/1 -> P Control/5(High Limit)
  Constant1/1 -> P Control/3(GAIN)
  SETPT(6)/1 -> P Control/1(SETPT)
  Unit Delay/1 -> P Control/2(XMV_OLD)
  P Control/1(XMV_NEW) -> XMV(6)/1, Unit Delay/1
  Sampling interval/1 -> P Control/Action
  Constant3/1 -> Sampling interval/1
  XMEAS/1 -> P Control/4(XMEAS)

== system Simulink_TEP/Subsystem/Braatz/ 2/CONTROL 13 ==
  XMEAS(23) : Inport
  Constant : Constant  Value=SETPT13
  Constant1 : Constant  Value=GAIN13
  Constant2 : Constant  Value=TAUI13
  Constant3 : Constant  Value=HIGH13
  Constant5 : Constant  Value=SI13
  Constant6 : Constant  Value=HIGH3
  PI Control Setpoint : mylib/Braatz Control/PI Control Setpoint  SystemSampleTime=-1  VariantActivationTime=update diagram  AllowFlexibleInterface=on  Latency=0  AutoFrameSizeCalculation=off
  Sampling interval : mylib/Braatz Control/Sampling interval  SystemSampleTime=-1  VariantActivationTime=update diagram  AllowFlexibleInterface=on  Latency=0  AutoFrameSizeCalculation=off
  Unit Delay : UnitDelay  InitialCondition=SETPT3  SampleTime=-1  HasFrameUpgradeWarning=on
  Unit Delay1 : UnitDelay  SampleTime=-1  HasFrameUpgradeWarning=on
  SETPT(3) : Outport  VectorParamsAs1DForOutWhenUnconnected=off
  wires:
  Sampling interval/1 -> PI Control Setpoint/Action
  Constant/1 -> PI Control Setpoint/1
  XMEAS(23)/1 -> PI Control Setpoint/2
  PI Control Setpoint/1 -> SETPT(3)/1, Unit Delay/1
  Constant2/1 -> PI Control Setpoint/8
  Constant5/1 -> PI Control Setpoint/7, Sampling interval/1
  Constant1/1 -> PI Control Setpoint/6
  Constant3/1 -> PI Control Setpoint/3
  Unit Delay/1 -> PI Control Setpoint/4
  Constant6/1 -> PI Control Setpoint/5
  PI Control Setpoint/2 -> Unit Delay1/1
  Unit Delay1/1 -> PI Control Setpoint/9

== system Simulink_TEP/Subsystem/Braatz/ 2/CONTROL 3 ==
  XMEAS(1) : Inport
  SETPT(3) : Inport  Port=2
  Constant1 : Constant  Value=GAIN3
  Constant2 : Constant  Value=HIGH3
  Constant3 : Constant  Value=SI3
  P Control : mylib/Braatz Control/P Control  SystemSampleTime=-1  VariantActivationTime=update diagram  AllowFlexibleInterface=on  Latency=0  AutoFrameSizeCalculation=off
  Sampling interval : mylib/Braatz Control/Sampling interval  SystemSampleTime=-1  VariantActivationTime=update diagram  AllowFlexibleInterface=on  Latency=0  AutoFrameSizeCalculation=off
  Unit Delay : UnitDelay  InitialCondition=XMV3_0  SampleTime=-1  HasFrameUpgradeWarning=on
  Unit Delay1 : UnitDelay  SampleTime=-1  HasFrameUpgradeWarning=on
  XMV(3) : Outport  VectorParamsAs1DForOutWhenUnconnected=off
  wires:
  Constant2/1 -> P Control/5
  Constant1/1 -> P Control/3
  SETPT(3)/1 -> P Control/1
  Unit Delay/1 -> P Control/2
  XMEAS(1)/1 -> P Control/4
  P Control/1 -> XMV(3)/1, Unit Delay/1
  Sampling interval/1 -> P Control/Action
  Constant3/1 -> Sampling interval/1
  P Control/2 -> Unit Delay1/1
  Unit Delay1/1 -> P Control/6

== system Simulink_TEP/Subsystem/Braatz/ 3/CONTROL 17 ==
  XMEAS(8) : Inport
  Constant : Constant  Value=SETPT17
  Constant1 : Constant  Value=GAIN17
  Constant2 : Constant  Value=TAUI17
  Constant3 : Constant  Value=HIGH17
  Constant5 : Constant  Value=SI17
  Constant6 : Constant  Value=HIGH4
  PI Control Setpoint : mylib/Braatz Control/PI Control Setpoint  SystemSampleTime=-1  VariantActivationTime=update diagram  AllowFlexibleInterface=on  Latency=0  AutoFrameSizeCalculation=off
  Sampling interval : mylib/Braatz Control/Sampling interval  SystemSampleTime=-1  VariantActivationTime=update diagram  AllowFlexibleInterface=on  Latency=0  AutoFrameSizeCalculation=off
  Unit Delay : UnitDelay  InitialCondition=SETPT4  SampleTime=-1  HasFrameUpgradeWarning=on
  Unit Delay1 : UnitDelay  SampleTime=-1  HasFrameUpgradeWarning=on
  SETPT(4) : Outport  VectorParamsAs1DForOutWhenUnconnected=off
  wires:
  Sampling interval/1 -> PI Control Setpoint/Action
  Constant/1 -> PI Control Setpoint/1
  XMEAS(8)/1 -> PI Control Setpoint/2
  PI Control Setpoint/1 -> SETPT(4)/1, Unit Delay/1
  Constant2/1 -> PI Control Setpoint/8
  Constant5/1 -> PI Control Setpoint/7, Sampling interval/1
  Constant1/1 -> PI Control Setpoint/6
  Constant3/1 -> PI Control Setpoint/3
  Unit Delay/1 -> PI Control Setpoint/4
  Constant6/1 -> PI Control Setpoint/5
  PI Control Setpoint/2 -> Unit Delay1/1
  Unit Delay1/1 -> PI Control Setpoint/9

== system Simulink_TEP/Subsystem/Braatz/ 3/CONTROL 4 ==
  XMEAS(4) : Inport
  SETPT(4) : Inport  Port=2
  Constant1 : Constant  Value=GAIN4
  Constant2 : Constant  Value=HIGH4
  Constant3 : Constant  Value=SI4
  P Control : mylib/Braatz Control/P Control  SystemSampleTime=-1  VariantActivationTime=update diagram  AllowFlexibleInterface=on  Latency=0  AutoFrameSizeCalculation=off
  Sampling interval : mylib/Braatz Control/Sampling interval  SystemSampleTime=-1  VariantActivationTime=update diagram  AllowFlexibleInterface=on  Latency=0  AutoFrameSizeCalculation=off
  Unit Delay : UnitDelay  InitialCondition=XMV4_0  SampleTime=-1  HasFrameUpgradeWarning=on
  Unit Delay1 : UnitDelay  SampleTime=-1  HasFrameUpgradeWarning=on
  XMV(4) : Outport  VectorParamsAs1DForOutWhenUnconnected=off
  wires:
  Constant2/1 -> P Control/5
  Constant1/1 -> P Control/3
  SETPT(4)/1 -> P Control/1
  Unit Delay/1 -> P Control/2
  XMEAS(4)/1 -> P Control/4
  P Control/1 -> XMV(4)/1, Unit Delay/1
  Sampling interval/1 -> P Control/Action
  Constant3/1 -> Sampling interval/1
  P Control/2 -> Unit Delay1/1
  Unit Delay1/1 -> P Control/6

== system Simulink_TEP/Subsystem/Braatz/ 4/CONTROL 5 ==
  XMEAS(5) : Inport
  Constant1 : Constant  Value=GAIN5
  Constant2 : Constant  Value=HIGH5
  Constant3 : Constant  Value=SI5
  Constant4 : Constant  Value=SETPT5
  Constant5 : Constant  Value=TAUI5
  PI Control : mylib/Braatz Control/PI Control  SystemSampleTime=-1  VariantActivationTime=update diagram  AllowFlexibleInterface=on  Latency=0  AutoFrameSizeCalculation=off
  Sampling interval : mylib/Braatz Control/Sampling interval  SystemSampleTime=-1  VariantActivationTime=update diagram  AllowFlexibleInterface=on  Latency=0  AutoFrameSizeCalculation=off
  Unit Delay : UnitDelay  InitialCondition=XMV5_0  SampleTime=-1  HasFrameUpgradeWarning=on
  Unit Delay1 : UnitDelay  SampleTime=-1  HasFrameUpgradeWarning=on
  XMV(5) : Outport  VectorParamsAs1DForOutWhenUnconnected=off
  wires:
  Constant2/1 -> PI Control/4
  Constant1/1 -> PI Control/5
  Unit Delay/1 -> PI Control/1
  XMEAS(5)/1 -> PI Control/3
  PI Control/1 -> Unit Delay/1, XMV(5)/1
  Sampling interval/1 -> PI Control/Action
  Constant3/1 -> PI Control/6, Sampling interval/1
  Constant4/1 -> PI Control/2
  Constant5/1 -> PI Control/7
  PI Control/2 -> Unit Delay1/1
  Unit Delay1/1 -> PI Control/8

== system Simulink_TEP/Subsystem/Braatz/ 5/CONTROL 7 ==
  XMEAS(12) : Inport
  Constant1 : Constant  Value=GAIN7
  Constant2 : Constant  Value=HIGH7
  Constant3 : Constant  Value=SI7
  Constant4 : Constant  Value=SETPT7
  P Control : mylib/Braatz Control/P Control  SystemSampleTime=-1  VariantActivationTime=update diagram  AllowFlexibleInterface=on  Latency=0  AutoFrameSizeCalculation=off
  Sampling interval : mylib/Braatz Control/Sampling interval  SystemSampleTime=-1  VariantActivationTime=update diagram  AllowFlexibleInterface=on  Latency=0  AutoFrameSizeCalculation=off
  Unit Delay : UnitDelay  InitialCondition=XMV7_0  SampleTime=-1  HasFrameUpgradeWarning=on
  Unit Delay1 : UnitDelay  SampleTime=-1  HasFrameUpgradeWarning=on
  XMV(7) : Outport  VectorParamsAs1DForOutWhenUnconnected=off
  wires:
  Constant2/1 -> P Control/5
  Constant1/1 -> P Control/3
  Unit Delay/1 -> P Control/2
  XMEAS(12)/1 -> P Control/4
  P Control/1 -> Unit Delay/1, XMV(7)/1
  Sampling interval/1 -> P Control/Action
  Constant3/1 -> Sampling interval/1
  Constant4/1 -> P Control/1
  P Control/2 -> Unit Delay1/1
  Unit Delay1/1 -> P Control/6

== system Simulink_TEP/Subsystem/Braatz/ 6/CONTROL 8 ==
  XMEAS(15) : Inport
  Constant1 : Constant  Value=GAIN8
  Constant2 : Constant  Value=HIGH8
  Constant3 : Constant  Value=SI8
  Constant4 : Constant  Value=SETPT8
  P Control : mylib/Braatz Control/P Control  SystemSampleTime=-1  VariantActivationTime=update diagram  AllowFlexibleInterface=on  Latency=0  AutoFrameSizeCalculation=off
  Sampling interval : mylib/Braatz Control/Sampling interval  SystemSampleTime=-1  VariantActivationTime=update diagram  AllowFlexibleInterface=on  Latency=0  AutoFrameSizeCalculation=off
  Unit Delay : UnitDelay  InitialCondition=XMV8_0  SampleTime=-1  HasFrameUpgradeWarning=on
  Unit Delay1 : UnitDelay  SampleTime=-1  HasFrameUpgradeWarning=on
  XMV(8) : Outport  VectorParamsAs1DForOutWhenUnconnected=off
  wires:
  Constant2/1 -> P Control/5
  Constant1/1 -> P Control/3
  Unit Delay/1 -> P Control/2
  XMEAS(15)/1 -> P Control/4
  P Control/1 -> Unit Delay/1, XMV(8)/1
  Sampling interval/1 -> P Control/Action
  Constant3/1 -> Sampling interval/1
  Constant4/1 -> P Control/1
  P Control/2 -> Unit Delay1/1
  Unit Delay1/1 -> P Control/6

== system Simulink_TEP/Subsystem/Braatz/ 7/CONTROL 11 ==
  XMEAS(17) : Inport
  Constant1 : Constant  Value=GAIN11
  Constant2 : Constant  Value=HIGH11
  Constant3 : Constant  Value=SI11
  Constant4 : Constant  Value=SETPT11
  Constant5 : Constant  Value=TAUI11
  PI Control : mylib/Braatz Control/PI Control  SystemSampleTime=-1  VariantActivationTime=update diagram  AllowFlexibleInterface=on  Latency=0  AutoFrameSizeCalculation=off
  Sampling interval : mylib/Braatz Control/Sampling interval  SystemSampleTime=-1  VariantActivationTime=update diagram  AllowFlexibleInterface=on  Latency=0  AutoFrameSizeCalculation=off
  Unit Delay : UnitDelay  InitialCondition=XMV11_0  SampleTime=-1  HasFrameUpgradeWarning=on
  Unit Delay1 : UnitDelay  SampleTime=-1  HasFrameUpgradeWarning=on
  XMV(11) : Outport  VectorParamsAs1DForOutWhenUnconnected=off
  wires:
  Constant2/1 -> PI Control/4
  Constant1/1 -> PI Control/5
  Unit Delay/1 -> PI Control/1
  XMEAS(17)/1 -> PI Control/3
  PI Control/1 -> Unit Delay/1, XMV(11)/1
  Sampling interval/1 -> PI Control/Action
  Constant3/1 -> PI Control/6, Sampling interval/1
  Constant4/1 -> PI Control/2
  Constant5/1 -> PI Control/7
  PI Control/2 -> Unit Delay1/1
  Unit Delay1/1 -> PI Control/8

== system Simulink_TEP/Subsystem/Braatz/ 8/CONTROL 10 ==
  XMEAS(21) : Inport
  SETPT(10) : Inport  Port=2
  Constant1 : Constant  Value=GAIN10
  Constant2 : Constant  Value=HIGH10
  Constant3 : Constant  Value=SI10
  Constant4 : Constant  Value=TAUI10
  PI Control : mylib/Braatz Control/PI Control  SystemSampleTime=-1  VariantActivationTime=update diagram  AllowFlexibleInterface=on  Latency=0  AutoFrameSizeCalculation=off
  Sampling interval : mylib/Braatz Control/Sampling interval  SystemSampleTime=-1  VariantActivationTime=update diagram  AllowFlexibleInterface=on  Latency=0  AutoFrameSizeCalculation=off
  Unit Delay : UnitDelay  InitialCondition=XMV10_0  SampleTime=-1  HasFrameUpgradeWarning=on
  Unit Delay1 : UnitDelay  SampleTime=-1  HasFrameUpgradeWarning=on
  XMV(10) : Outport  VectorParamsAs1DForOutWhenUnconnected=off
  wires:
  SETPT(10)/1 -> PI Control/2
  Unit Delay/1 -> PI Control/1
  XMEAS(21)/1 -> PI Control/3
  PI Control/1 -> XMV(10)/1, Unit Delay/1
  Sampling interval/1 -> PI Control/Action
  Constant3/1 -> PI Control/6, Sampling interval/1
  Constant2/1 -> PI Control/4
  Constant1/1 -> PI Control/5
  Constant4/1 -> PI Control/7
  PI Control/2 -> Unit Delay1/1
  Unit Delay1/1 -> PI Control/8

== system Simulink_TEP/Subsystem/Braatz/ 8/CONTROL 18 ==
  XMEAS(9) : Inport
  Constant : Constant  Value=SETPT18
  Constant1 : Constant  Value=GAIN18
  Constant2 : Constant  Value=TAUI18
  Constant3 : Constant  Value=HIGH18
  Constant5 : Constant  Value=SI18
  Constant6 : Constant  Value=HIGH10
  PI Control Setpoint : mylib/Braatz Control/PI Control Setpoint  SystemSampleTime=-1  VariantActivationTime=update diagram  AllowFlexibleInterface=on  Latency=0  AutoFrameSizeCalculation=off
  Sampling interval : mylib/Braatz Control/Sampling interval  SystemSampleTime=-1  VariantActivationTime=update diagram  AllowFlexibleInterface=on  Latency=0  AutoFrameSizeCalculation=off
  Unit Delay : UnitDelay  InitialCondition=SETPT10  SampleTime=-1  HasFrameUpgradeWarning=on
  Unit Delay1 : UnitDelay  SampleTime=-1  HasFrameUpgradeWarning=on
  SETPT(10) : Outport  VectorParamsAs1DForOutWhenUnconnected=off
  wires:
  Sampling interval/1 -> PI Control Setpoint/Action
  Constant/1 -> PI Control Setpoint/1
  XMEAS(9)/1 -> PI Control Setpoint/2
  PI Control Setpoint/1 -> SETPT(10)/1, Unit Delay/1
  Constant2/1 -> PI Control Setpoint/8
  Constant5/1 -> PI Control Setpoint/7, Sampling interval/1
  Constant1/1 -> PI Control Setpoint/6
  Constant3/1 -> PI Control Setpoint/3
  Unit Delay/1 -> PI Control Setpoint/4
  Constant6/1 -> PI Control Setpoint/5
  PI Control Setpoint/2 -> Unit Delay1/1
  Unit Delay1/1 -> PI Control Setpoint/9
